simulink model "xobserver"  (R2018a)
settings: Solver=ode45  StartTime=0.0  StopTime=24.5344
model workspace (MAT data in the model file):
  control.time = [141836678 141936659 142036839 142136747 142236726 142336833 142436727 142536732 142636755 142736950 142836707 142936893 ... (334 elements, 334x1)]
  control.ut = [0.6636588 0.6723409 0.6993658 0.6606792 0.6636723 0.6418326 0.6306298 0.6112502 0.5904683 0.5719165 0.5606404 0.5478745 ... (334 elements, 334x1)]
  control.ur = [-0.01929347 0.008807245 0.01339692 -0.01049517 -0.001550599 0.008109259 -0.002307277 -0.02206673 -0.04954416 -0.03543702 -0.04225481 -0.020684 ... (334 elements, 334x1)]
  control.up = [-0.003905352 -0.06342705 -0.08035815 -0.125074 -0.1411634 -0.1212279 -0.08798932 -0.04043218 -0.01298343 -0.03998712 -0.01606168 0.01761314 ... (334 elements, 334x1)]
  control.uy = [0.01393014 0.02556528 0.0444511 0.06274941 0.08221094 0.1058014 0.1303824 0.1531353 0.1686528 0.1777345 0.1843161 0.1906641 ... (334 elements, 334x1)]
  input.time = [137013148 137105522 137113114 137205498 137213142 137305502 137313143 137385536 137393177 137505497 137513125 137605502 ... (665 elements, 665x1)]
  input.signals.values = [8.71560944851e-05 -0.000263895544732 0.000265805954332 0.000300014003894 0.000591371497193 0.000529778841884 0.00684193504836 0.00668914061072 0.00254694811157 -0.00143805981445 -0.0136823182856 -0.0178010839904 ... (3325 elements, 665x5)]
  l = 3335
  l1 = 2807
  l2 = 674
  lcontrol = 334
  lt = 665
  output.time_lapsed = [141.842951 141.85293 141.86295 141.87293 141.88275 141.892944 141.902979 141.912936 141.922988 141.932751 141.942933 141.952953 ... (3335 elements, 1x3335)]
  output.euler_angles = [-0.00584184250158 -0.00582752686931 -0.00599777389745 -0.00620480390784 -0.00702123060925 -0.00776037504077 -0.00872918351285 -0.00978595795539 -0.0111794014087 -0.0126574335944 -0.00142848656261 -0.00317215629721 ... (10005 elements, 3335x3)]
  output.velocity_NED = [0.000184390535147 -0.00149610425919 -0.00223334883079 -0.000713157886509 -0.000766576163703 -0.00387684468628 -0.00670103088207 -0.00734005889528 0.0450059481743 0.0433575925328 0.0369973932984 0.0353518917006 ... (10005 elements, 3335x3)]
  output.position_NED = [8.41007051927e-07 -1.10001369642e-05 -2.61641403349e-05 -5.80451134531e-05 -8.88303667884e-05 -0.000121087190081 -0.000167699484482 -0.000220541528278 0.000446765501289 0.000888026171248 0.00119146179416 0.00155632925884 ... (10005 elements, 3335x3)]
  output.gyro_bias = [0 0 0 0 0 -3.65006890493e-17 -1.35602048461e-16 -1.35602048461e-16 -1.35602048461e-16 -1.35602048461e-16 -1.29991687392e-11 -1.29991687392e-11 ... (10005 elements, 3335x3)]
  output.accel_bias = [0 0 0 0 0 2.11086099686e-12 4.55721928734e-12 4.55721928734e-12 4.55721928734e-12 4.55721928734e-12 4.05772026724e-09 4.05772026724e-09 ... (10005 elements, 3335x3)]
  output.mag_NED = [0.156941993728 0.156941993728 0.156941993728 0.156941993728 0.156941993728 0.156941993728 0.156941993728 0.156941993728 0.156941993728 0.156941993728 0.168048584891 0.168048584891 ... (10005 elements, 3335x3)]
  output.mag_XYZ = [0 0 0 0 0 0 0 0 0 0 7.18989582303e-05 7.18989582303e-05 ... (10005 elements, 3335x3)]
  output.wind_NE = [0 0 0 0 0 0 0 0 0 0 0 0 ... (6670 elements, 3335x2)]
  output.dt = 0.0100139388739
  output.state_variance = []
  output.innovations.hgt_time_lapsed = [141.842951 141.88275 141.892944 141.982921 141.992932 142.08294 142.092946 142.182941 142.192973 142.282959 142.292952 142.382985 ... (381 elements, 1x381)]
  output.innovations.hgtInnov = [0.0839809268476 0.229196406766 0.205751842392 0.303062243401 0.275619937826 0.107674031475 0.0959693356033 -0.130355896388 -0.127822401048 -0.41012568378 -0.391486749275 -0.790016186459 ... (381 elements, 1x381)]
  output.innovations.hgtInnovVar = [2.25001089431 2.22248717759 2.20032667516 2.18365244656 2.16851124171 2.16024739358 2.14918417282 2.14157166145 2.1330485463 2.13566461103 2.12867825897 2.12041975372 ... (381 elements, 1x381)]
  output.innovations.vel_time_lapsed = [141.912936 142.112885 142.312858 142.512954 142.712935 142.91298 143.112962 143.312946 143.512926 143.712963 143.912756 144.112953 ... (269 elements, 1x269)]
  output.innovations.vel_innov = [0 -0.297209341318 -0.234893183313 0.621979504496 0.585229738761 0.320789024533 0.543137141152 -0.287873063317 -0.110706247412 -0.120646162284 -0.163914163339 -0.156973194534 ... (807 elements, 269x3)]
  output.innovations.vel_innov_var = [0.469842876227 0.720238945838 0.830910393732 0.685047383519 0.501853614365 0.408912593373 0.407605860139 0.431058610766 0.482687363738 0.438846363961 0.5397992737 0.457930605243 ... (807 elements, 269x3)]
  output.innovations.pos_time_lapsed = [141.912936 142.112885 142.312858 142.512954 142.712935 142.91298 143.112962 143.312946 143.512926 143.712963 143.912756 144.112953 ... (269 elements, 1x269)]
  output.innovations.posInnov = [0 0.0491974588037 0.230709594745 0.184905242738 0.167459180481 0.101502552362 0.0367561551374 0.0977833320685 0.0809762867801 0.0711637532904 0.014143071259 -0.0506785133148 ... (538 elements, 269x2)]
  output.innovations.posInnovVar = [3.43693035561 2.16772400471 1.87173245778 1.66498743326 1.50327332619 1.42962486409 1.39471999692 1.36145559416 1.34582786285 1.33384351194 1.32706102372 1.32075964401 ... (538 elements, 269x2)]
  output.innovations.magLength = [0.406783726321 0.404023514167 0.409106343143 0.403358401425 0.401103477921 0.401529575498 0.405513255024 0.404251159553 0.402288453724 0.400761774624 0.40280019861 0.401722541065 ... (499 elements, 1x499)]
  output.innovations.mag_time_lapsed = [141.932751 142.032945 142.132938 142.232929 142.332941 142.432932 142.532989 142.632926 142.732976 142.832927 142.932939 143.032947 ... (499 elements, 1x499)]
  output.innovations.magInnov = [-0.0216978085871 -0.00268007195522 -0.00117321200832 -0.00610558646204 0.00333705984515 0.00882426915741 0.0189814854375 0.0190678898943 0.0235752652886 0.0232611770385 0.016992221986 0.0090804125995 ... (1497 elements, 499x3)]
  output.innovations.magInnovVar = [0.258794912157 0.00486619229406 0.00369420266798 0.00330597340814 0.00310507731597 0.00298704091331 0.00291656896492 0.00285730490122 0.00282339292197 0.00278570180343 0.00275564295281 0.0027328155134 ... (1497 elements, 499x3)]
  output.magFuseMethod = 1
  output.state_variances = [0.0100000049606 0.0100000133987 0.0100000222965 0.0100000369864 0.0100000586546 0.0100000699069 0.0100000712503 0.0100001052347 0.00946907698392 0.00946875606614 0.00920147105253 0.00920018099078 ... (80040 elements, 3335x24)]
  output.euler_variances = [0.0400039517326 0.0400028754196 0.0400019391425 0.0400010107041 0.0400004548436 0.0400005118133 0.0400014359189 0.0400032586352 0.0373806026767 0.0373842845766 0.0288751536704 0.0288658130855 ... (10005 elements, 3335x3)]
  output1.time_lapsed = [141.845249 141.855211 141.868043 141.878032 141.890201 141.902979 141.91522 141.928036 141.940194 141.952953 141.965268 141.97806 ... (2807 elements, 1x2807)]
  output1.euler_angles = [-0.00951294730114 -0.00920735413542 -0.00959414339571 -0.00994393705528 -0.010521564041 -0.011647107134 -0.0130811250416 -0.0146303708573 -0.00412926564345 -0.000658426850056 -0.00341025687951 -0.00560376389235 ... (8421 elements, 2807x3)]
  output1.velocity_NED = [-0.0072911566562 -0.00056320239423 -0.00599141921129 -0.00781011846976 -0.00340602573042 -0.00843145399503 -0.00579798145971 0.0420528050757 0.0353949993433 0.0327194391449 0.0257099146215 0.0275019940691 ... (8421 elements, 2807x3)]
  output1.position_NED = [-2.7591005686e-06 -1.30820701188e-05 -4.96121897726e-05 -9.92463455975e-05 -0.00016395292104 -0.000253049012508 -0.000337992859002 0.000567219774502 0.000962159350865 0.00136365783405 0.00172496581561 0.00207670269858 ... (8421 elements, 2807x3)]
  output1.gyro_bias = [0 0 0 0 0 3.66956010595e-17 3.66956010595e-17 3.66956010595e-17 -1.65351262305e-11 -2.58330802929e-11 -2.58330802929e-11 -2.58330802929e-11 ... (8421 elements, 2807x3)]
  output1.accel_bias = [0 0 0 0 0 -2.863554223e-12 -2.863554223e-12 -2.863554223e-12 8.92121800719e-09 1.31770985729e-08 1.31770985729e-08 1.31770985729e-08 ... (8421 elements, 2807x3)]
  output1.mag_NED = [0.142821731677 0.142821731677 0.142821731677 0.142821731677 0.142821731677 0.142821731677 0.142821731677 0.142821731677 0.155865095223 0.156626447973 0.156626447973 0.156626447973 ... (8421 elements, 2807x3)]
  output1.mag_XYZ = [0 0 0 0 0 0 0 0 6.68508938599e-05 9.92420284271e-05 9.92420284271e-05 9.92420284271e-05 ... (8421 elements, 2807x3)]
  output1.wind_NE = [0 0 0 0 0 0 0 0 0 0 0 0 ... (5614 elements, 2807x2)]
  output1.dt = 0.0118970477374
  output1.state_variance = []
  output1.innovations.hgt_time_lapsed = [141.845249 141.890201 141.97806 141.990198 142.085223 142.190199 142.282959 142.295243 142.382985 142.39524 142.488014 142.588071 ... (354 elements, 1x354)]
  output1.innovations.hgtInnov = [0.0838516250697 0.228590399935 0.324900749293 0.293448248561 0.125892020073 -0.101976149729 -0.378595380533 -0.359633927634 -0.790647133282 -0.752872406699 -0.721308093143 -0.507136442603 ... (354 elements, 1x354)]
  output1.innovations.hgtInnovVar = [2.250006258 2.22235849858 2.20086827611 2.18275885504 2.17102298448 2.15785926786 2.15164710168 2.14199175512 2.13080925513 2.12332037282 2.1211761498 2.11635546671 ... (354 elements, 1x354)]
  output1.innovations.vel_time_lapsed = [141.91522 142.108024 142.120194 142.307836 142.32019 142.512954 142.712935 142.905269 142.918026 143.118041 143.310203 143.322936 ... (241 elements, 1x241)]
  output1.innovations.vel_innov = [0 0.223218097268 0.0782198451563 -0.0393523739168 -0.0433557704498 -0.203349495356 -0.34765933246 -0.200230428814 -0.114918626504 0.0855181776422 0.0746144886608 0.0649662439355 ... (723 elements, 241x3)]
  output1.innovations.vel_innov_var = [0.272173120267 0.538621896396 0.361911220085 0.458595479609 0.340214614374 0.384175012924 0.377701241913 0.338057524276 0.282340326669 0.294483582163 0.302252086366 0.279799571511 ... (723 elements, 241x3)]
  output1.innovations.pos_time_lapsed = [141.91522 142.108024 142.120194 142.307836 142.32019 142.512954 142.712935 142.905269 142.918026 143.118041 143.310203 143.322936 ... (241 elements, 1x241)]
  output1.innovations.posInnov = [0 0.0632397957884 0.0390651551697 0.0525898457077 0.0397411304575 0.0574354246896 0.0722490444019 0.0429978352649 0.0424160452693 0.00174344416799 0.0340691516275 0.0217481136763 ... (482 elements, 241x2)]
  output1.innovations.posInnovVar = [1.3378425785 1.09085761544 0.990291720466 0.930554249845 0.894935065735 0.876195925891 0.864424296467 0.855487155994 0.840054201323 0.836604797944 0.834255837168 0.82367983954 ... (482 elements, 241x2)]
  output1.innovations.magLength = [0.400263663102 0.400263663102 0.400036248358 0.400036248358 0.401321566826 0.401321566826 0.399753674154 0.398794433261 0.403352203415 0.403352203415 0.399899987497 0.396532470297 ... (520 elements, 1x520)]
  output1.innovations.mag_time_lapsed = [141.928036 141.940194 142.028024 142.04022 142.130194 142.142953 142.235257 142.332941 142.430196 142.440195 142.538033 142.638022 ... (520 elements, 1x520)]
  output1.innovations.magInnov = [-0.0218360458745 -0.00320172206261 0.000231112091682 -0.00135151361159 -0.000791157058328 -0.00218987587495 -0.00328524669996 0.00569991094716 0.00873818670504 0.00883340674107 0.012821010392 0.0194479404538 ... (1560 elements, 520x3)]
  output1.innovations.magInnovVar = [0.258292995633 0.00487295593552 0.00370586363577 0.00331058171518 0.00311582973031 0.00299386461659 0.0029139515405 0.0028471454507 0.00280556088545 0.00277192269911 0.00274394116584 0.00272306224028 ... (1560 elements, 520x3)]
  output1.magFuseMethod = 1
  output1.state_variances = [0.0100000068787 0.0100000139265 0.0100000288991 0.0100000458389 0.0100000848112 0.0100001034535 0.0100001623673 0.00901773095881 0.00878565435361 0.00870964747549 0.00870687653565 0.00870446462992 ... (67368 elements, 2807x24)]
  output1.euler_variances = [0.0400008554254 0.0400014858603 0.0400027705482 0.0400045778478 0.0400083841847 0.0400137405887 0.0400211908957 0.0353164135129 0.0263847265996 0.0232072072811 0.0231918507424 0.0231719196773 ... (8421 elements, 2807x3)]
  pitch = [-0.00601170594305 0.00114522514384 0.0125445164557 0.0260129427859 0.0413526501937 0.0511756269945 0.0373024628261 0.0532548324432 0.0752374412467 0.0870367972512 0.0703790408797 0.0642023494021 ... (665 elements, 665x1)]
  pitch1 = [0.00235222572609 0.0162413418271 0.0237914073903 0.038703711523 0.0528926975341 0.0693959637901 0.125700648169 0.149036541994 0.168586162345 0.181978559157 0.17648303704 0.173940572128 ... (665 elements, 665x1)]
  roll = [-0.00280308900026 -0.0093555701281 -0.00623960724973 -0.00965013944258 -0.0144960083544 -0.0165739618303 -0.0413451111402 -0.0417587932814 -0.039753610855 -0.0382742391951 -0.0474672160662 -0.0523524236581 ... (665 elements, 665x1)]
  roll1 = [-0.00508976540984 -0.0128769177256 -0.00573808802069 -0.00803683640664 -0.0148569990238 -0.0135250113299 0.00757283220458 0.0108108566268 0.0110824245139 0.0117467287189 0.0115391118445 0.00812049366445 ... (665 elements, 665x1)]
  rtk_P = [0 0 0.00725817699424 0.00725817699424 -4.192609801e-16 -4.192609801e-16 0.00725817698288 0.00725817698288 -6.06069014419e-17 -6.06069014419e-17 0.00725817697152 0.00725817697152 ... (2022 elements, 674x3)]
  simin.time_lapsed = [141.842951 141.85293 141.86295 141.87293 141.88275 141.892944 141.902979 141.912936 141.922988 141.932751 141.942933 141.952953 ... (3335 elements, 1x3335)]
  simin.euler_angles = [-0.00584184250158 -0.00582752686931 -0.00599777389745 -0.00620480390784 -0.00702123060925 -0.00776037504077 -0.00872918351285 -0.00978595795539 -0.0111794014087 -0.0126574335944 -0.00142848656261 -0.00317215629721 ... (10005 elements, 3335x3)]
  simin.velocity_NED = [0.000184390535147 -0.00149610425919 -0.00223334883079 -0.000713157886509 -0.000766576163703 -0.00387684468628 -0.00670103088207 -0.00734005889528 0.0450059481743 0.0433575925328 0.0369973932984 0.0353518917006 ... (10005 elements, 3335x3)]
  simin.position_NED = [8.41007051927e-07 -1.10001369642e-05 -2.61641403349e-05 -5.80451134531e-05 -8.88303667884e-05 -0.000121087190081 -0.000167699484482 -0.000220541528278 0.000446765501289 0.000888026171248 0.00119146179416 0.00155632925884 ... (10005 elements, 3335x3)]
  simin.gyro_bias = [0 0 0 0 0 -3.65006890493e-17 -1.35602048461e-16 -1.35602048461e-16 -1.35602048461e-16 -1.35602048461e-16 -1.29991687392e-11 -1.29991687392e-11 ... (10005 elements, 3335x3)]
  simin.accel_bias = [0 0 0 0 0 2.11086099686e-12 4.55721928734e-12 4.55721928734e-12 4.55721928734e-12 4.55721928734e-12 4.05772026724e-09 4.05772026724e-09 ... (10005 elements, 3335x3)]
  simin.mag_NED = [0.156941993728 0.156941993728 0.156941993728 0.156941993728 0.156941993728 0.156941993728 0.156941993728 0.156941993728 0.156941993728 0.156941993728 0.168048584891 0.168048584891 ... (10005 elements, 3335x3)]
  simin.mag_XYZ = [0 0 0 0 0 0 0 0 0 0 7.18989582303e-05 7.18989582303e-05 ... (10005 elements, 3335x3)]
  simin.wind_NE = [0 0 0 0 0 0 0 0 0 0 0 0 ... (6670 elements, 3335x2)]
  simin.dt = 0.0100139388739
  simin.state_variance = []
  simin.innovations.hgt_time_lapsed = [141.842951 141.88275 141.892944 141.982921 141.992932 142.08294 142.092946 142.182941 142.192973 142.282959 142.292952 142.382985 ... (381 elements, 1x381)]
  simin.innovations.hgtInnov = [0.0839809268476 0.229196406766 0.205751842392 0.303062243401 0.275619937826 0.107674031475 0.0959693356033 -0.130355896388 -0.127822401048 -0.41012568378 -0.391486749275 -0.790016186459 ... (381 elements, 1x381)]
  simin.innovations.hgtInnovVar = [2.25001089431 2.22248717759 2.20032667516 2.18365244656 2.16851124171 2.16024739358 2.14918417282 2.14157166145 2.1330485463 2.13566461103 2.12867825897 2.12041975372 ... (381 elements, 1x381)]
  simin.innovations.vel_time_lapsed = [141.912936 142.112885 142.312858 142.512954 142.712935 142.91298 143.112962 143.312946 143.512926 143.712963 143.912756 144.112953 ... (269 elements, 1x269)]
  simin.innovations.vel_innov = [0 -0.297209341318 -0.234893183313 0.621979504496 0.585229738761 0.320789024533 0.543137141152 -0.287873063317 -0.110706247412 -0.120646162284 -0.163914163339 -0.156973194534 ... (807 elements, 269x3)]
  simin.innovations.vel_innov_var = [0.469842876227 0.720238945838 0.830910393732 0.685047383519 0.501853614365 0.408912593373 0.407605860139 0.431058610766 0.482687363738 0.438846363961 0.5397992737 0.457930605243 ... (807 elements, 269x3)]
  simin.innovations.pos_time_lapsed = [141.912936 142.112885 142.312858 142.512954 142.712935 142.91298 143.112962 143.312946 143.512926 143.712963 143.912756 144.112953 ... (269 elements, 1x269)]
  simin.innovations.posInnov = [0 0.0491974588037 0.230709594745 0.184905242738 0.167459180481 0.101502552362 0.0367561551374 0.0977833320685 0.0809762867801 0.0711637532904 0.014143071259 -0.0506785133148 ... (538 elements, 269x2)]
  simin.innovations.posInnovVar = [3.43693035561 2.16772400471 1.87173245778 1.66498743326 1.50327332619 1.42962486409 1.39471999692 1.36145559416 1.34582786285 1.33384351194 1.32706102372 1.32075964401 ... (538 elements, 269x2)]
  simin.innovations.magLength = [0.406783726321 0.404023514167 0.409106343143 0.403358401425 0.401103477921 0.401529575498 0.405513255024 0.404251159553 0.402288453724 0.400761774624 0.40280019861 0.401722541065 ... (499 elements, 1x499)]
  simin.innovations.mag_time_lapsed = [141.932751 142.032945 142.132938 142.232929 142.332941 142.432932 142.532989 142.632926 142.732976 142.832927 142.932939 143.032947 ... (499 elements, 1x499)]
  simin.innovations.magInnov = [-0.0216978085871 -0.00268007195522 -0.00117321200832 -0.00610558646204 0.00333705984515 0.00882426915741 0.0189814854375 0.0190678898943 0.0235752652886 0.0232611770385 0.016992221986 0.0090804125995 ... (1497 elements, 499x3)]
  simin.innovations.magInnovVar = [0.258794912157 0.00486619229406 0.00369420266798 0.00330597340814 0.00310507731597 0.00298704091331 0.00291656896492 0.00285730490122 0.00282339292197 0.00278570180343 0.00275564295281 0.0027328155134 ... (1497 elements, 499x3)]
  simin.magFuseMethod = 1
  simin.state_variances = [0.0100000049606 0.0100000133987 0.0100000222965 0.0100000369864 0.0100000586546 0.0100000699069 0.0100000712503 0.0100001052347 0.00946907698392 0.00946875606614 0.00920147105253 0.00920018099078 ... (80040 elements, 3335x24)]
  simin.euler_variances = [0.0400039517326 0.0400028754196 0.0400019391425 0.0400010107041 0.0400004548436 0.0400005118133 0.0400014359189 0.0400032586352 0.0373806026767 0.0373842845766 0.0288751536704 0.0288658130855 ... (10005 elements, 3335x3)]
  t = [85.2681087899 153.847078989 135.937655107 145.710208503 139.738803374 143.646452387 141.245887466 142.795164057 141.986419874 142.477492231 142.340892456 142.389396391 ... (674 elements, 674x1)]
  temp = [0.000186264650653 -0.000333016556148 0.00127742410264 0.00224038281138 0.00429726594319 -0.00123745127094 -0.0498635877438 -0.0654781132175 -0.0797628012916 -0.0994190421594 -0.130389530625 -0.157448428987 ... (674 elements, 674x1)]
  time = [137013148 137105522 137113114 137205498 137213142 137305502 137313143 137385536 137393177 137505497 137513125 137605502 ... (665 elements, 665x1)]
  tout = [0; 40; 80; 120; 160; 200; 240; 280; 320; 360; 400; 440; 480; 520; 560; 600; 640; 680; 720; 760; 800; 840; 880; 920; 960; 1000; 1040; 1080; 1120; 1160; 1200; 1240; 1280; 1320; 1360; 1400; 1440; 1480; 1520; 1560; 1600; 1640; 1680; 1720; 1760; 1800; 1840; 1880; 1920; 1960; 2000]
  ups = [-0.00390798864963 -0.0343320965106 -0.0636578539957 -0.075087173802 -0.0805963166531 -0.0991310672402 -0.125807682301 -0.141612416937 -0.141039897482 -0.132345709554 -0.120718475957 -0.105525554245 ... (665 elements, 665x1)]
  urs = [-0.0193064957453 -0.00988556947443 0.00896900324588 0.0192245887848 0.0131872654637 -0.000864770461033 -0.0106332547779 -0.00981483295256 -0.00119475892361 0.00693320512295 0.00799889781381 0.00317561720843 ... (665 elements, 665x1)]
  uts = [0.664106860951 0.749481484877 0.672099541838 0.648171853238 0.700691335264 0.708512249166 0.659850468498 0.640879189244 0.664961763399 0.668205140062 0.640989688844 0.625700347079 ... (665 elements, 665x1)]
  uys = [0.0139395447601 0.0198481563309 0.0256425224772 0.0339606547853 0.0446716994275 0.0544470884218 0.06301463774 0.0718767917399 0.0826736407 0.0943232231429 0.10641126735 0.11853603151 ... (665 elements, 665x1)]
  x = [8.71560944851e-05 -0.000263895544732 0.000265805954332 0.000300014003894 0.000591371497193 0.000529778841884 0.00684193504836 0.00668914061072 0.00254694811157 -0.00143805981445 -0.0136823182856 -0.0178010839904 ... (665 elements, 665x1)]
  x1 = [8.54283814042e-05 -0.000351541918258 0.000561343727981 0.00122062991294 0.00226118745505 0.0017878063312 -0.0048216263535 -0.0106732543262 -0.0180693220189 -0.0278330591582 -0.0298109986026 -0.0413157469741 ... (665 elements, 665x1)]
  x_av = [8.62922379446e-05 -0.000307718731495 0.000413574841157 0.000760321958416 0.00142627947612 0.00115879258654 0.00101015434743 -0.00199205685772 -0.00776118695365 -0.0146355594863 -0.0217466584441 -0.0295584154823 ... (665 elements, 665x1)]
  xt = [-6.06069014419e-17 0.00725817697152 0.00725817697152 -5.47955244547e-11 -5.47955244547e-11 -5.57118682784e-11 -5.57118682784e-11 -0.00725817702815 -0.00725817702815 -0.0145163542274 -0.0145163542274 -0.0290327088019 ... (665 elements, 665x1)]
  y = [4.71199364932e-05 -0.000202451032641 0.00110205359743 0.00274075291804 0.00386317545071 0.0039759501557 0.0111320604636 0.0200674919449 0.0256167559869 0.0328388617799 0.00902856975366 0.0187732326011 ... (665 elements, 665x1)]
  y1 = [0.000186264650653 -0.000333016556148 0.00127742410264 0.00224038281138 0.00429726594319 -0.00123745127094 -0.0498635877438 -0.0654781132175 -0.0797628012916 -0.0994190421594 -0.130389530625 -0.157448428987 ... (665 elements, 665x1)]
  y_av = [0.000116692293573 -0.000267733794395 0.00118973885004 0.00249056786471 0.00408022069695 0.00136924944238 -0.0193657636401 -0.0227053106363 -0.0270730226523 -0.0332900901898 -0.0606804804357 -0.0693375981928 ... (665 elements, 665x1)]
  yaw = [0.551630744054 0.985953522054 0.860467849076 0.912170384354 0.864267212524 0.877979115519 0.85252446167 0.850917442274 0.835099319744 0.825993656962 0.8192363021 0.809230396231 ... (665 elements, 665x1)]
  yaw1 = [0.524311158471 0.914078236382 0.795656408279 0.841193934159 0.796803282272 0.809519389357 0.787366234758 0.785910630038 0.771945888619 0.763168855651 0.757543515422 0.745155737898 ... (665 elements, 665x1)]
  yt = [2.07646400074e-15 -8.22783768201e-10 -8.22783768201e-10 -0.0111218847698 -0.0111218847698 -0.0222437696223 -0.0222437696223 -0.0333656546197 -0.0333656546197 -0.0444875400883 -0.0444875400883 -0.0667313107556 ... (665 elements, 665x1)]
  z = [-0.0994666679592 -0.214162644666 -0.215226967159 -0.256145303395 -0.292239651406 -0.309925352113 -0.350361829325 -0.36096245045 -0.394865238248 -0.398678408621 -0.417742992449 -0.417553654594 ... (674 elements, 674x1)]
  z1 = [-0.103229820714 -0.203136396463 -0.194407590044 -0.247819005734 -0.277075354685 -0.291884441153 -0.321788426104 -0.334001860067 -0.367445284083 -0.368818531247 -0.415153871284 -0.416306471083 ... (674 elements, 674x1)]
libraries: dspmathops x3
(part 1 of 2)
settings Model: Creator=hamahuss_admin  LastModifiedBy=hussein

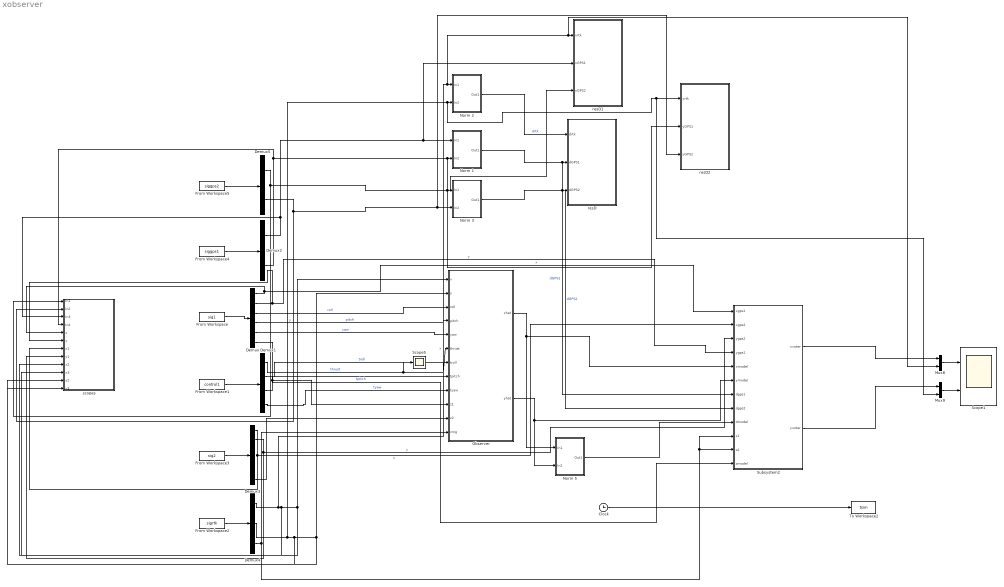
== system xobserver ==
  Clock : Clock
  Demux : Demux  Outputs=6
  Demux1 : Demux
  Demux2 : Demux  Outputs=2
  Demux3 : Demux  Outputs=6
  Demux4 : Demux  Outputs=3
  Demux5 : Demux  Outputs=2
  From Workspace : FromWorkspace  VariableName=sig1
  From Workspace1 : FromWorkspace  VariableName=control1
  From Workspace2 : FromWorkspace  VariableName=sigrtk
  From Workspace3 : FromWorkspace  VariableName=sig2
  From Workspace4 : FromWorkspace  VariableName=siggps1
  From Workspace5 : FromWorkspace  VariableName=siggps2
  Mux8 : Mux  Inputs=2
  Mux9 : Mux  Inputs=2
  Norm 1 : Subsystem
  Norm 2 : Subsystem
  Norm 3 : Subsystem
  Norm 5 : Subsystem
  "Observer " : Subsystem
  Scope1 : Scope  NumInputPorts=2
  Scope5 : Scope
  Subsystem2 : Subsystem
  To Workspace2 : ToWorkspace  VariableName=tsim  SampleTime=-1
  resD : Subsystem
  resD1 : Subsystem
  resD2 : Subsystem
  "scopes " : Subsystem
  wires:
  From Workspace/1 -> Demux/1
  From Workspace1/1 -> Demux1/1
  From Workspace3/1 -> Demux3/1
  From Workspace2/1 -> Demux4/1
  Norm 2/1(Out1) -> resD/1(drtk)  "drtk"
  Norm 1/1(Out1) -> Subsystem2/7("dgps1 "), resD/2(dGPS1)  "dGPS1"
  Norm 3/1(Out1) -> Subsystem2/8(dgps2), resD/3(dGPS2)  "dGPS2"
  Demux4/2 -> Mux9/2, resD2/1(yrtk), Norm 2/2(In2), "scopes "/11(y2), "scopes "/12(y3), "Observer "/2(y)  "y"
  Demux4/1 -> Mux8/2, resD1/1(xrtk), Norm 2/1(In1), "scopes "/9(x2), "scopes "/10(x3), "Observer "/1(x)  "x"
  From Workspace4/1 -> Demux2/1
  From Workspace5/1 -> Demux5/1
  Demux2/1 -> "scopes "/3(In3), resD1/2(xGPS1), Norm 1/1(In1)
  Demux2/2 -> "scopes "/4(In4), resD2/2(yGPS1), Norm 1/2(In2)
  Demux5/1 -> "scopes "/1(In1), resD1/3(xGPS2), Norm 3/1(In1)
  Demux5/2 -> "scopes "/2(In2), Norm 3/2(In2), resD2/3(yGPS2)
  Demux/3 -> "Observer "/3(roll)  "roll"
  Demux/4 -> "Observer "/4(pitch)  "pitch"
  Demux/5 -> "Observer "/5(yaw)  "yaw"
  Demux1/1 -> Scope5/1, "Observer "/6(thrust)  "thrust"
  Demux1/2 -> "Observer "/7(troll)  "troll"
  Demux1/3 -> "Observer "/8(tpitch)  "tpitch"
  Demux1/4 -> "Observer "/9(tyaw)  "tyaw"
  "Observer "/1(xhat) -> Norm 5/1(In1), Subsystem2/5("xmodel ")
  "Observer "/2(yhat) -> Subsystem2/6("ymodel "), Norm 5/2(In2)
  Mux9/1 -> Scope1/2
  Mux8/1 -> Scope1/1
  Subsystem2/1("xvoter ") -> Mux8/1
  Subsystem2/2(yvoter) -> Mux9/1
  Norm 5/1(Out1) -> Subsystem2/9("dmodel ")
  Demux/6 -> Subsystem2/12("zmodel "), "Observer "/10(z1)
  Demux3/6 -> "Observer "/11(z2)
  Demux4/3 -> Subsystem2/10("z1 "), Subsystem2/11(z2), "Observer "/12("zrng ")
  Demux/1 -> Subsystem2/1("xgps1 "), "scopes "/5(x)  "x"
  Demux/2 -> Subsystem2/4(ygps1), "scopes "/6(y)  "y"
  Demux3/1 -> Subsystem2/2("xgps2 "), "scopes "/7(x1)  "x"
  Demux3/2 -> Subsystem2/3("ygps2 "), "scopes "/8(y1)  "y"
  Clock/1 -> To Workspace2/1
